simulink model "RotorVirtualPlantModel_DigitalControl"  (R2022b)
settings: Solver=VariableStepAuto  StartTime=0.0  StopTime=2  RelTol=1e-3
values from neighbouring files (symbols this model uses):
  b = 4.425*1e-6    (= 4.425e-06)    [rotor_control_ownparams.m]
  C_d_den = cell2mat(C_d.den)    [rotor_control_ownparams.m]
  C_d_num = cell2mat(C_d.num)    [rotor_control_ownparams.m]
  J_rotor = J_rodc+J_motor    (= 1.8053e-05)    [rotor_control_ownparams.m]
  K_m = 0.025463    [rotor_control_ownparams.m]
  L = 0    [rotor_control_ownparams.m]
  R = 6    [rotor_control_ownparams.m]
  Ts = 0.001    [rotor_control_ownparams.m]
  V_s = 10.5    [rotor_control_ownparams.m]
settings Model: Creator=TC Tsao  LastModifiedBy=pruth
settings SolverCC: AlgebraicLoopSolver=TrustRegion
settings DebuggingCC: UnconnectedInputMsg=warning  UnconnectedOutputMsg=warning  UnconnectedLineMsg=warning  SFMachineParentedDataDiag=warning
settings ModelReferenceCC: EnableRefExpFcnMdlSchedulingChecks=on
settings RTWCC: DLArmComputeVersion=19.05

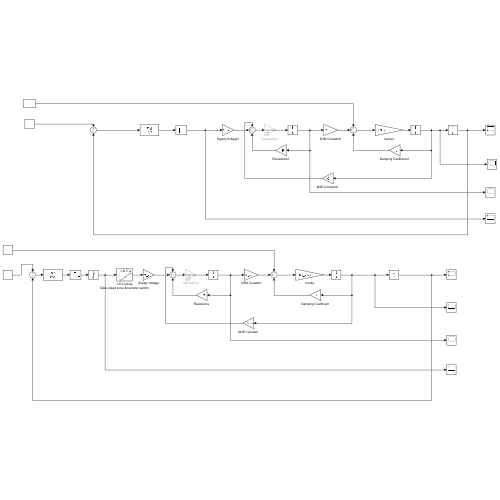
[thumbnail: Simulink's stored preview of the top-level diagram]
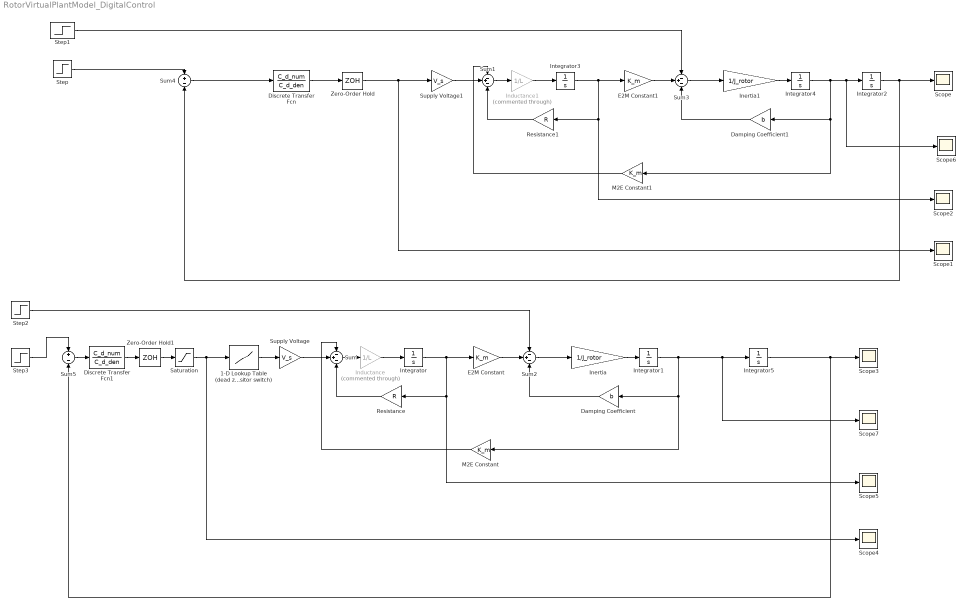
== system RotorVirtualPlantModel_DigitalControl ==
  1-D Lookup Table (dead zone & transitor switch) : Lookup_n-D  NumberOfTableDimensions=1  BreakpointsForDimension1=[-1,-0.96,-0.1,-0.06,-0.04,0,0.04,0.06,0.1,0.96,1]  Table=[-10.8,-10.8,-2,-1,-0,0,0,1,2,10.8,10.8]/V_s  InternalRulePriority=Speed  RndMeth=Simplest
  Damping Coefficient : Gain  Gain=b
  Damping Coefficient1 : Gain  Gain=b
  Discrete Transfer Fcn : DiscreteTransferFcn  Numerator=C_d_num  Denominator=C_d_den  SampleTime=Ts
  Discrete Transfer Fcn1 : DiscreteTransferFcn  Numerator=C_d_num  Denominator=C_d_den  SampleTime=Ts
  E2M Constant : Gain  Gain=K_m
  E2M Constant1 : Gain  Gain=K_m
  Inductance : Gain  Commented=through  Gain=1/L
  Inductance1 : Gain  Commented=through  Gain=1/L
  Inertia : Gain  Gain=1/J_rotor
  Inertia1 : Gain  Gain=1/J_rotor
  Integrator{,1..5} (6 alike) : Integrator
  M2E Constant : Gain  Gain=K_m
  M2E Constant1 : Gain  Gain=K_m
  Resistance : Gain  Gain=R
  Resistance1 : Gain  Gain=R
  Saturation : Saturate  UpperLimit=1  LowerLimit=-1
  Scope{,1..7} (8 alike) : Scope
  Step : Step  Time=0  SampleTime=0
  Step1 : Step  After=0.05  SampleTime=0
  Step2 : Step  After=0.05  SampleTime=0
  Step3 : Step  Time=0  SampleTime=0
  Sum{,1..3} (4 alike) : Sum  Inputs=-+-
  Sum4 : Sum  Inputs=+-
  Sum5 : Sum  Inputs=+-
  Supply Voltage : Gain  Gain=V_s
  Supply Voltage1 : Gain  Gain=V_s
  Zero-Order Hold : ZeroOrderHold  SampleTime=-1
  Zero-Order Hold1 : ZeroOrderHold  SampleTime=-1
  wires:
  Supply Voltage/1 -> Sum/2
  Sum2/1 -> Inertia/1
  Inertia/1 -> Integrator1/1
  Sum/1 -> Inductance/1
  Sum1/1 -> Inductance1/1
  M2E Constant1/1 -> Sum1/1
  Inductance1/1 -> Integrator3/1
  Resistance/1 -> Sum/3
  Step2/1 -> Sum2/1
  Resistance1/1 -> Sum1/3
  E2M Constant1/1 -> Sum3/2
  Integrator/1 -> E2M Constant/1, Scope5/1, Resistance/1
  M2E Constant/1 -> Sum/1
  Supply Voltage1/1 -> Sum1/2
  Damping Coefficient/1 -> Sum2/3
  Sum3/1 -> Inertia1/1
  Inertia1/1 -> Integrator4/1
  Integrator3/1 -> E2M Constant1/1, Scope2/1, Resistance1/1
  Inductance/1 -> Integrator/1
  Damping Coefficient1/1 -> Sum3/3
  Step1/1 -> Sum3/1
  1-D Lookup Table (dead zone & transitor switch)/1 -> Supply Voltage/1
  E2M Constant/1 -> Sum2/2
  Step/1 -> Sum4/1
  Integrator4/1 -> Scope6/1, Integrator2/1, M2E Constant1/1, Damping Coefficient1/1
  Zero-Order Hold/1 -> Scope1/1, Supply Voltage1/1
  Sum4/1 -> Discrete Transfer Fcn/1
  Sum5/1 -> Discrete Transfer Fcn1/1
  Step3/1 -> Sum5/1
  Integrator1/1 -> Scope7/1, Integrator5/1, M2E Constant/1, Damping Coefficient/1
  Zero-Order Hold1/1 -> Saturation/1
  Discrete Transfer Fcn/1 -> Zero-Order Hold/1
  Discrete Transfer Fcn1/1 -> Zero-Order Hold1/1
  Integrator2/1 -> Sum4/2, Scope/1
  Integrator5/1 -> Sum5/2, Scope3/1
  Saturation/1 -> 1-D Lookup Table (dead zone & transitor switch)/1, Scope4/1
